simulink model "commHW3slx"  (R2020b)
settings: Solver=VariableStepAuto  StartTime=0.0  StopTime=0.4  RelTol=1e-3
undefined symbols (not defined in the file or in its folder): DiscIntNeverNeededParam
libraries: dspsigops x1, simulink x1
settings Model: Creator=Acer  LastModifiedBy=Acer

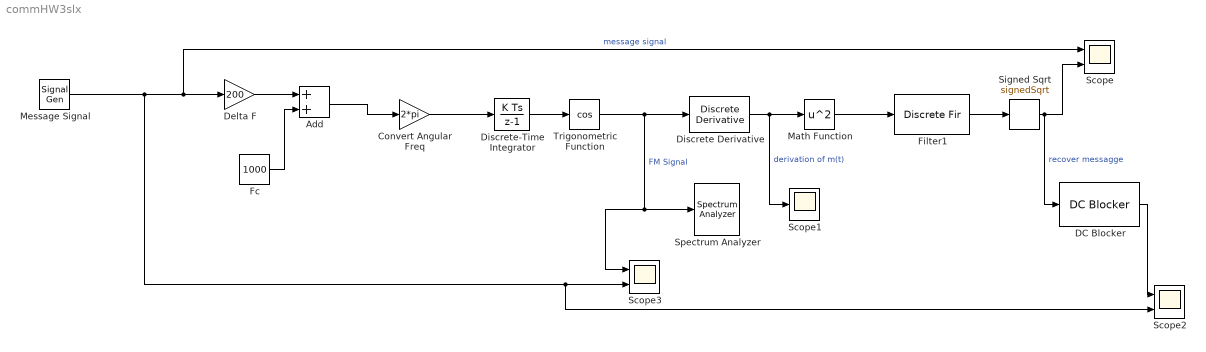
== system commHW3slx ==
  Add : Sum
  Convert Angular Freq : Gain  Gain=2*pi
  DC Blocker : dspsigops/DC Blocker  Algorithm=FIR  NormalizedBandwidth=0.0001  Length=20000  Order=8  SimulateUsing=Code generation
      settings: SourceProductName=DSP System Toolbox
  Delta F : Gain  Gain=200
  Discrete Derivative : simulink/Discrete/Discrete Derivative  gainval=1e-3  ICPrevScaledInput=0.0  OutMin=[]  OutMax=[]  OutDataType=fixdt(1, 16)  OutScaling=2^-10  DoSatur=off
  Discrete-Time Integrator : DiscreteIntegrator  gainval=1  SampleTime=1e-5  ICPrevOutput=DiscIntNeverNeededParam  ICPrevScaledInput=DiscIntNeverNeededParam
  Fc : Constant  Value=1000
  Filter1 : DiscreteFir  Tag=BlockMethodSubSystem  Coefficients=[0.000112763886687097841 5.25887244708979576e-05 6.43223399680057175e-05 7.74316063993968806e-05 9.19397712165416936e-05 0.000107882517517894432 0.000125198623332952938 0.000143878501653206477 0.000163872182044479987 0.000185185429020982866 0.000207675342998350879 0.000231209284559730287 0.00025562669051162792 0.0002809333130029432 0.000306791208994216245 0.000332920575245950162 0.000359277434456304235 0.000385338763741785353 0.000410986520409636674 0.000435793822854463624 0.000459438790476235847 0.000481493885730547493 0.00050157365661377437 0.00051923799103312674 0.000534016044584766656 0.000545415291303876252 0.000552967545655343412 0.000556180286730491866 0.000554510066155081984 0.000547497334634638663 0.000534603736925841778 0.000515305986481587363 0.000489160540276478489 0.000455646134289950018 0.000414342085659391633 0.000364794894471180545 0.000306644378162700061 0.000239527218016726782 0.000163147843097470894 7.72532546034955135e-05 -1.83389533453550514e-05 -0.000123771484358511366 -0.000239088465953546673 -0.000364261392813968582 -0.000499215754337983472 -0.000643746368284181308 -0.000797582895908662166 -0.00096036170517031891 -0.00113160549244915626 -0.00131075998644286174 -0.00149714112736521344 -0.00168999105286141149 -0.00188841873889327534 -0.00209144973379003741 -0.0022980015433630035 -0.00250689828117563705 -0.00271684474778451524 -0.00292647686395760111 -0.00313432613637016667 -0.00333883396701411921 -0.00353838060238625789 -0.00373125645503572401 -0.00391569927511920077 -0.00408989019928887067 -0.00425196659450294192 -0.00440003697872141074 -0.00453217211269357594 -0.00464645010747429671 -0.00474093983403112845 -0.00481372805330595836 -0.0048629246808926975 -0.00488669155585777157 -0.00488322656240367838 -0.00485081320847054187 -0.00478781108518112203 -0.00469267272213452942 -0.00456396676038133952 -0.00440038145582840635 -0.00420074957051409792 -0.00396404615077351058 -0.00368941028700677486 -0.00337615754786202817 -0.00302377793664173212 -0.00263196056664353507 -0.00220059412658714241 -0.00172977386042333045 -0.00121980439935619103 -0.000671220966530613615 -8.47694506477737373e-05 0.00053857270196730402 0.001197607257897749 0.00189090927130507267 0.00261683224423323989 0.00337351365831478796 0.00415887258257745425 0.00497062839974910225 0.00580630264785578394 0.00666322485256308147 0.00753855138996988462 0.00842927679752190732 0.00933224348510018967 0.0102441586832942022 0.0111616156597206442 0.0120811012082031669 0.0129990245752276135 0.0139117289981526907 0.0148155183833198652 0.0157066680018462732 0.0165814524334452346 0.0174361679046162246 0.0182671465653657591 0.0190707819730259916 0.0198435516574727681 0.0205820347297030713 0.0212829325333130162 0.0219430927143542259 0.0225595233207224674 0.0231294105118661532 0.0236501393752912084 0.0241193092504946166 0.0245347467514829103 0.0248945171540714445 0.0251969428746055546 0.0254406071284052487 0.0256243654060155299 0.0257473542668271854 0.025808995012285979 0.025808995012285979 0.0257473542668271854 0.0256243654060155299 0.0254406071284052487 0.0251969428746055546 0.0248945171540714445 0.0245347467514829103 0.0241193092504946166 0.0236501393752912084 0.0231294105118661532 0.0225595233207224674 0.0219430927143542259 0.0212829325333130162 0.0205820347297030713 0.0198435516574727681 0.0190707819730259916 0.0182671465653657591 0.0174361679046162246 0.0165814524334452346 0.0157066680018462732 0.0148155183833198652 0.0139117289981526907 0.0129990245752276135 0.0120811012082031669 0.0111616156597206442 0.0102441586832942022 0.00933224348510018967 0.00842927679752190732 0.00753855138996988462 0.00666322485256308147 0.00580630264785578394 0.00497062839974910225 0.00415887258257745425 0.00337351365831478796 0.00261683224423323989 0.00189090927130507267 0.001197607257897749 0.00053857270196730402 -8.47694506477737373e-05 -0.000671220966530613615 -0.00121980439935619103 -0.00172977386042333045 -0.00220059412658714241 -0.00263196056664353507 -0.00302377793664173212 ...(+1968 chars)]  InputProcessing=Columns as channels (frame based)
  Math Function : Math  Operator=square  SaturateOnIntegerOverflow=on
  Message Signal : SignalGenerator  WaveForm=square  Frequency=10
  Scope : Scope  NumInputPorts=2
  Scope1 : Scope
  Scope2 : Scope  NumInputPorts=2
  Scope3 : Scope  NumInputPorts=2
  Signed Sqrt : Sqrt  Operator=signedSqrt  SaturateOnIntegerOverflow=on
  Spectrum Analyzer : SpectrumAnalyzer
  Trigonometric Function : Trigonometry  Operator=cos
  wires:
  Delta F/1 -> Add/1
  Fc/1 -> Add/2
  Add/1 -> Convert Angular Freq/1
  Convert Angular Freq/1 -> Discrete-Time Integrator/1
  Discrete-Time Integrator/1 -> Trigonometric Function/1
  Trigonometric Function/1 -> Discrete Derivative/1, Scope3/1, Spectrum Analyzer/1  "FM Signal"
  Discrete Derivative/1 -> Scope1/1, Math Function/1  "derivation of m(t)"
  Signed Sqrt/1 -> DC Blocker/1, Scope/2  "recover messagge"
  Math Function/1 -> Filter1/1
  Filter1/1 -> Signed Sqrt/1
  Message Signal/1 -> Scope2/2, Scope3/2, Scope/1, Delta F/1  "message signal"
  DC Blocker/1 -> Scope2/1
